simulink model "MASTER"  (R2024b)
settings: configuration reference "STM32H7_Config" (kept outside this file)
libraries: simulink x2
settings Model: DataDictionary=Master_Dictionary.sldd  EnableAccessToBaseWorkspace=off  TickDuration=2.0E-08  Creator=torni  LastModifiedBy=oxbro
settings ConfigSetRef: SourceName=STM32H7_Config

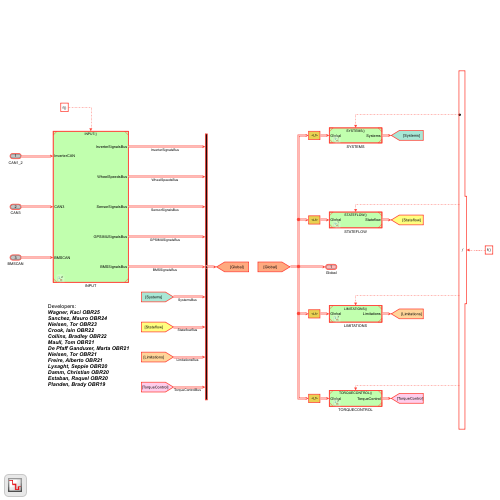
[thumbnail: Simulink's stored preview of the top-level diagram]
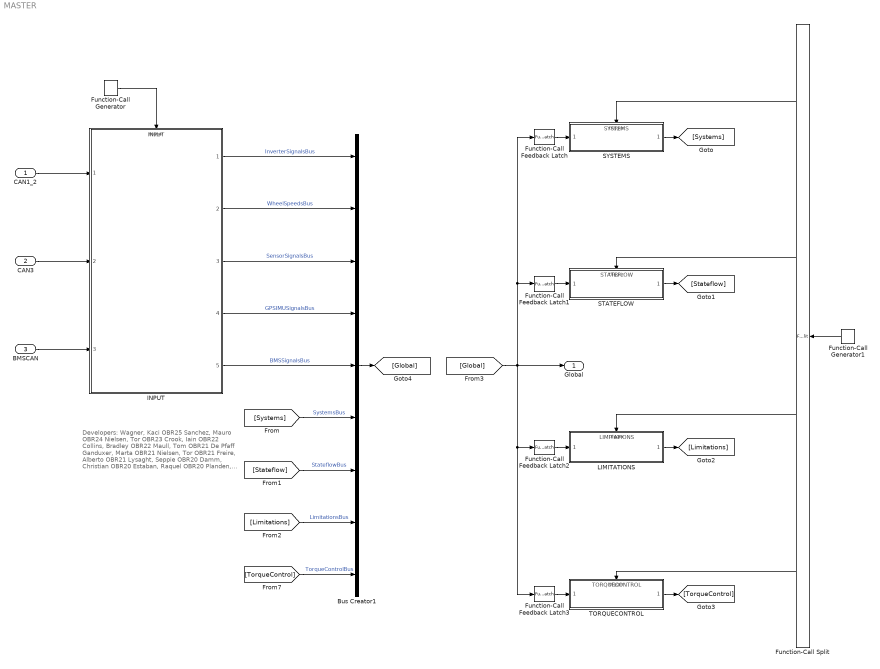
== system MASTER ==
  note: Developers:
      | Wagner, Kaci OBR25
      | Sanchez, Mauro OBR24
      | Nielsen, Tor OBR23
      | Crook, Iain OBR22
      | Collins, Bradley OBR22
      | Maull, Tom OBR21
      | De Pfaff Ganduxer, Marta OBR21
      | Nielsen, Tor OBR21
      | Freire, Alberto OBR21
      | Lysaght, Seppie OBR20
      | Damm, Christian OBR20
      | Estaban, Raquel OBR20
      | Planden, Brady OBR19
  CAN1_2 : Inport  OutDataTypeStr=Bus: CAN1_2Bus
  CAN3 : Inport  Port=2  OutDataTypeStr=Bus: CAN3Bus
  BMSCAN : Inport  Port=3  OutDataTypeStr=Bus: CAN4Bus
  Bus Creator1 : BusCreator  Inputs=9  OutDataTypeStr=Bus: Global
  Function-Call Feedback Latch{,1..3} (4 alike) : FunctionCallFeedbackLatch
  Function-Call Generator : simulink/Ports & Subsystems/Function-Call Generator  sample_time=-1  numberOfIterations=1  DisallowWideOutput=off
  Function-Call Generator1 : simulink/Ports & Subsystems/Function-Call Generator  sample_time=-1  numberOfIterations=1  DisallowWideOutput=off
  Function-Call Split : FunctionCallSplit  IconShape=distinctive  NumOutputPorts=4  OutputPortLayout=default
  INPUT : ModelReference  ModelNameDialog=INPUT  SimulationMode=Normal  ModelReferenceVersion=13.20  TriggerPortName=Trigger  TriggerPortTriggerType=function-call  TriggerPortStatesWhenEnabling=held
  LIMITATIONS : ModelReference  ModelNameDialog=LIMITATIONS  SimulationMode=Normal  ModelReferenceVersion=13.7  TriggerPortName=Trigger  TriggerPortTriggerType=function-call  TriggerPortStatesWhenEnabling=held
  STATEFLOW : ModelReference  ModelNameDialog=STATEFLOW  SimulationMode=Normal  ModelReferenceVersion=13.8  TriggerPortName=Trigger  TriggerPortTriggerType=function-call  TriggerPortStatesWhenEnabling=held
  SYSTEMS : ModelReference  ModelNameDialog=SYSTEMS  SimulationMode=Normal  ModelReferenceVersion=13.7  TriggerPortName=Trigger  TriggerPortTriggerType=function-call  TriggerPortStatesWhenEnabling=held
  TORQUECONTROL : ModelReference  ModelNameDialog=TORQUECONTROL  SimulationMode=Normal  ModelReferenceVersion=13.8  TriggerPortName=Trigger  TriggerPortTriggerType=function-call  TriggerPortStatesWhenEnabling=held
  Global : Outport  OutDataTypeStr=Bus: Global  VectorParamsAs1DForOutWhenUnconnected=off
  wires:
  INPUT/1 -> Bus Creator1/1  "InverterSignalsBus"
  INPUT/2 -> Bus Creator1/2  "WheelSpeedsBus"
  INPUT/3 -> Bus Creator1/3  "SensorSignalsBus"
  INPUT/4 -> Bus Creator1/4  "GPSIMUSignalsBus"
  [Global] -> Global/1, Function-Call Feedback Latch/1, Function-Call Feedback Latch1/1, Function-Call Feedback Latch3/1, Function-Call Feedback Latch2/1
  SYSTEMS/1 -> [Systems]
  [Systems] -> Bus Creator1/6  "SystemsBus"
  Function-Call Feedback Latch/1 -> SYSTEMS/1
  Function-Call Feedback Latch1/1 -> STATEFLOW/1
  STATEFLOW/1 -> [Stateflow]
  [Stateflow] -> Bus Creator1/7  "StateflowBus"
  Function-Call Feedback Latch2/1 -> LIMITATIONS/1
  LIMITATIONS/1 -> [Limitations]
  [Limitations] -> Bus Creator1/8  "LimitationsBus"
  Function-Call Feedback Latch3/1 -> TORQUECONTROL/1
  TORQUECONTROL/1 -> [TorqueControl]
  INPUT/5 -> Bus Creator1/5  "BMSSignalsBus"
  [TorqueControl] -> Bus Creator1/9  "TorqueControlBus"
  Bus Creator1/1 -> [Global]
  Function-Call Generator1/1 -> Function-Call Split/1
  Function-Call Split/1 -> SYSTEMS/Trigger
  Function-Call Split/2 -> STATEFLOW/Trigger
  Function-Call Split/3 -> LIMITATIONS/Trigger
  Function-Call Split/4 -> TORQUECONTROL/Trigger
  CAN1_2/1 -> INPUT/1
  CAN3/1 -> INPUT/2
  BMSCAN/1 -> INPUT/3
  Function-Call Generator/1 -> INPUT/Trigger
